simulink library "gmp_simulink_utilities_src"  (R2022b)
settings: Solver=VariableStepAuto  StartTime=0.0  StopTime=10.0  RelTol=1e-3
settings Model: Creator=Javnson  LastModifiedBy=javnson

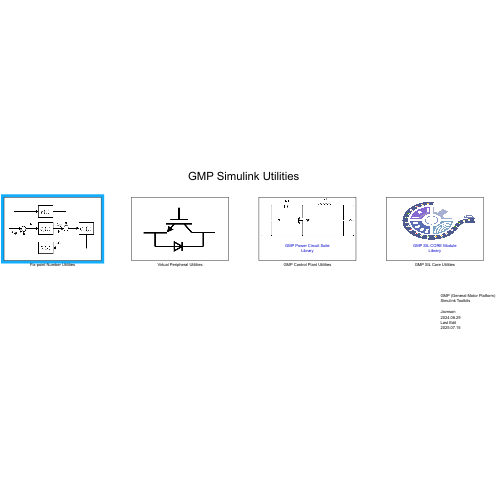
[thumbnail: Simulink's stored preview of the top-level diagram]
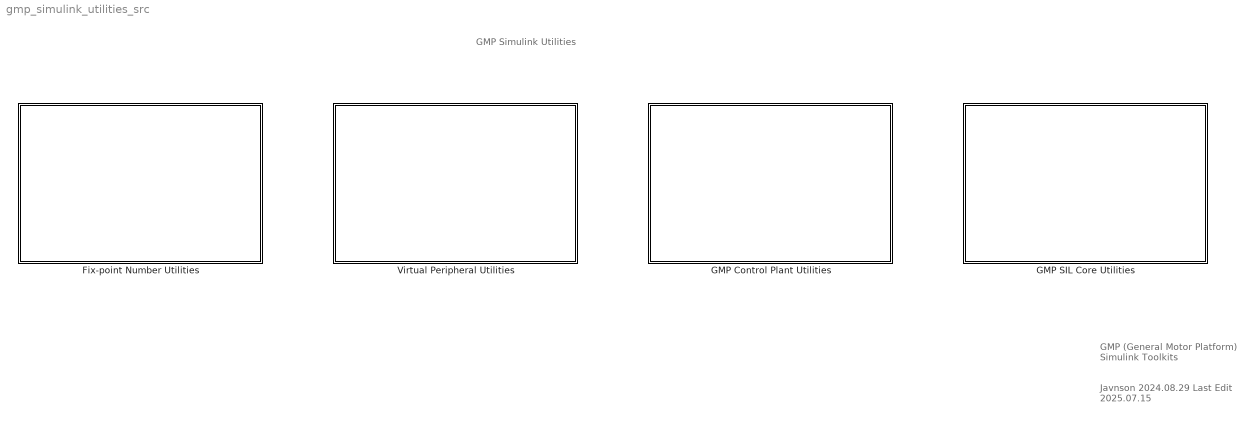
== system gmp_simulink_utilities_src ==
  note: GMP Simulink Utilities
  note: Javnson
      | 2024.08.29
      | Last Edit
      | 2025.07.15
  note: GMP (General Motor Platform)
      | Simulink Toolkits
  Fix-point Number Utilities : Subsystem
      settings: OpenFcn=gmp_fp_utilities
      mask Display: image(append(fileparts(which('gmp_simulink_utilities.slx')),'\icon\fp_lib_icon.png')); % 使用工具条上的 "编辑图像" 进行更改。
  GMP Control Plant Utilities : Subsystem
      settings: OpenFcn=gmp_std_model_pck
      mask Display:
      | image(append(fileparts(which('gmp_simulink_utilities.slx')),'\icon\power_suite.png'));
      | 
      | color('blue');
      | disp('\n\n\n\n\n\n\n\nGMP Power Circuit Suite\nLibrary');
  GMP SIL Core Utilities : Subsystem
      settings: OpenFcn=gmp_sil_core_pack
      mask Display:
      | image(append(fileparts(which('gmp_simulink_utilities.slx')),'\icon\GMP_Core.png'));
      | 
      | 
      | color('blue');
      | disp('\n\n\n\n\n\n\n\nGMP SIL CORE Module\nLibrary');
  Virtual Peripheral Utilities : Subsystem
      settings: OpenFcn=gmp_peripheral_utilities
      mask Display:
      | %fileparts(which('gmp_simulink_utilities.slx'))
      | 
      | image(append(fileparts(which('gmp_simulink_utilities.slx')),'\icon\Peripheral_lib_icon.png')); % 使用工具条上的 "编辑图像" 进行更改。

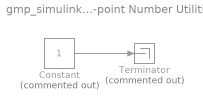
== system gmp_simulink_utilities_src/Fix-point Number Utilities ==
  Constant : Constant  Commented=on
  Terminator : Terminator  Commented=on
  wires:
  Constant/1 -> Terminator/1

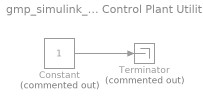
== system gmp_simulink_utilities_src/GMP Control Plant Utilities ==
  Constant : Constant  Commented=on
  Terminator : Terminator  Commented=on
  wires:
  Constant/1 -> Terminator/1

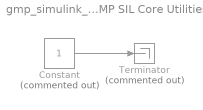
== system gmp_simulink_utilities_src/GMP SIL Core Utilities ==
  Constant : Constant  Commented=on
  Terminator : Terminator  Commented=on
  wires:
  Constant/1 -> Terminator/1

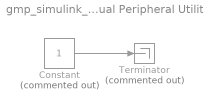
== system gmp_simulink_utilities_src/Virtual Peripheral Utilities ==
  Constant : Constant  Commented=on
  Terminator : Terminator  Commented=on
  wires:
  Constant/1 -> Terminator/1
